simulink model "smith_predictor_control"  (Simulink 5.0)
settings: Solver=FixedStepDiscrete  StartTime=0.0  StopTime=500.0  FixedStep=0.1  RelTol=1e-3
libraries: mathlib x9, execlib x2, genlib x2, modellib x2, reglib x1, analoglib x1, arclib x1
settings Model: LastModifiedBy=david  ExtModeTrigMode=oneshot  ExtModeArmWhenConnect=off  LimitDataPoints=off  BooleanDataType=off

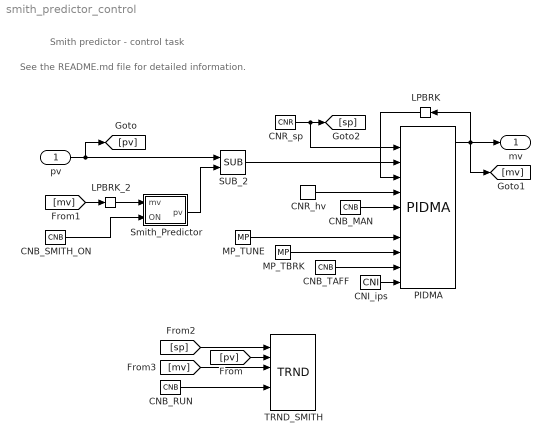
== system smith_predictor_control ==
  note: See the README.md file for detailed information.
  note: Smith predictor - control task
  pv : Inport  Port=1
  CNB_MAN : mathlib/CNB  YCN=off
  CNB_RUN : mathlib/CNB  YCN=on
  CNB_SMITH_ON : mathlib/CNB  YCN=off
  CNB_TAFF : mathlib/CNB  YCN=on
  CNI_ips : mathlib/CNI  icn=3
  CNR_hv : mathlib/CNR  ycn=0
  CNR_sp : mathlib/CNR  ycn=0
  LPBRK : execlib/LPBRK  Orientation=left
  LPBRK_2 : execlib/LPBRK
  MP_TBRK : genlib/MP  pwidth=1  BSTATE=off  RPTF=off
  MP_TUNE : genlib/MP  pwidth=1  BSTATE=off  RPTF=off
  PIDMA : reglib/PIDMA  irtype=6: PI  RACT=off  k=1  ti=5.5  td=0  nd=4  b=1  c=0  tt=1  hilim=1  lolim=-1  dz=0  icotype=1: Analog  ittype=6: PI  iainf=1: Static process  DGC=off  tdg=1  tn=2  amp=0.2  dy=0.1  ispeed=2: Normal (middle fast) CL  ipid=1: Parallel form
  SUB_2 : mathlib/SUB
  Smith_Predictor : Subsystem
      mask Type: REX sequence
  TRND_SMITH : arclib/TRND  n=3  l=1000  btype=8  ptype1=1: Store  ptype2=1: Store  ptype3=1: Store  ptype4=1: Store  pfac=1  afac=0  arc=0  id=1  Title=Trend Title  timesrc=1
  mv : Outport  Port=1
  wires:
  CNB_MAN/1 -> PIDMA/6
  CNB_RUN/1 -> TRND_SMITH/5
  CNB_SMITH_ON/1 -> Smith_Predictor/2(ON)
  CNB_TAFF/1 -> PIDMA/10
  CNI_ips/1 -> PIDMA/11
  CNR_hv/1 -> PIDMA/5
  CNR_sp/1 -> [sp], PIDMA/2
  [pv] -> TRND_SMITH/2
  [mv] -> LPBRK_2/1
  [sp] -> TRND_SMITH/1
  [mv] -> TRND_SMITH/3
  LPBRK/1 -> PIDMA/4
  LPBRK_2/1 -> Smith_Predictor/1(mv)
  MP_TBRK/1 -> PIDMA/9
  MP_TUNE/1 -> PIDMA/8
  PIDMA/1 -> [mv], LPBRK/1, mv/1
  SUB_2/1 -> PIDMA/3
  Smith_Predictor/1(pv) -> SUB_2/2
  pv/1 -> [pv], SUB_2/1

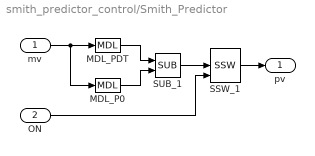
== system smith_predictor_control/Smith_Predictor ==
  mv : Inport  Port=1
  ON : Inport  Port=2
  MDL_P0 : modellib/MDL  k0=2.1  del=0  tau1=4.84  tau2=4.84  nmax=100
  MDL_PDT : modellib/MDL  k0=2.1  del=4.0  tau1=4.84  tau2=4.84  nmax=100
  SSW_1 : analoglib/SSW
  SUB_1 : mathlib/SUB
  pv : Outport  Port=1
  wires:
  MDL_P0/1 -> SUB_1/2
  MDL_PDT/1 -> SUB_1/1
  ON/1 -> SSW_1/3
  SSW_1/1 -> pv/1
  SUB_1/1 -> SSW_1/2
  mv/1 -> MDL_P0/1, MDL_PDT/1
